simulink model "SOF18d66"  (R2021a)
settings: Solver=VariableStepAuto  StartTime=0.0  StopTime=I_FF.time(end)  RelTol=1e-3
values from neighbouring files (symbols this model uses):
  betapol0 = 0.529567526316    [SOF18d66_setup.mat]
  equilInputs = [0 0 0 0 0 0 0 0 0 0 -1.36186383311e-26 -1.80160126662e-26 ... (15 elements, 1x15)]    [SOF18d66_setup.mat]
  equilOutputs = [-1399.7 -12059 -11927 -3903.5 -12061 -10328 8339.7 10474 2451.8 -17448 -1.80040840482e-24 -2.38174917622e-24 ... (1006 elements, 1x1006)]    [SOF18d66_setup.mat]
  equilVloop = 0.208271873891    [SOF18d66_setup.mat]
  EV_PS =     [SOF18d66_setup.mat]
  Input_struct =     [SOF18d66_setup.mat]
  IV_PS =     [SOF18d66_setup.mat]
  IVC_sat = 1000    [SOF18d66_setup.mat]
  li0 = 0.849401217093    [SOF18d66_setup.mat]
  nCirc = 10    [SOF18d66_setup.mat]
  nGaps = 31    [SOF18d66_setup.mat]
  nInVessel = 2    [SOF18d66_setup.mat]
  nMag = 957    [SOF18d66_setup.mat]
  PFC_sat = [1000 1300 1300 1000 1000 970 970 970 970 1000]    [SOF18d66_setup.mat]
undefined symbols (not defined in the file or in its folder): r_grid, R_grid, VS_contr, z_grid, Z_grid
libraries: cstblocks x6, JT60SA_Magnetic_Control x1
settings Model: Creator=adria  LastModifiedBy=adria

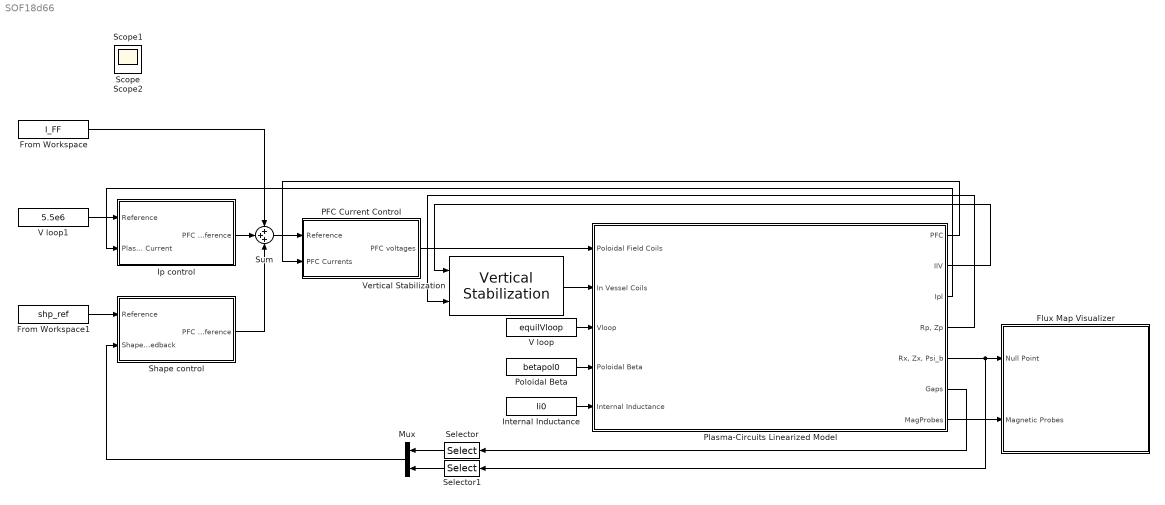
== system SOF18d66 ==
  Flux Map Visualizer : Subsystem  AncestorBlock=JT60SA_Magnetic_Control/Flux Map Visualizer  InitFcn=|  StartFcn=% fig_grid= figure()
      | addpath ./flux_grid_functions
      | [r_grid, z_grid, R_grid, Z_grid, F0, idxGrid] = initFluxGrid(Input_struct,y_np,y_type, mag, 0);
      mask Display:
      | image(['.' filesep 'images' filesep 'Grid.jpg'])
      | port_label('input',1,'Null Point');
      | port_label('input',2, 'Mag Probes');
  From Workspace : FromWorkspace  VariableName=I_FF
  From Workspace1 : FromWorkspace  VariableName=shp_ref
  Internal Inductance : Constant  Value=li0
  Ip control : Subsystem
  Mux : Mux  Inputs=2
  PFC Current Control : Subsystem  AncestorBlock=JT60SA_Magnetic_Control/PFC Current Control
      mask help: PF Coils Current Controller
      mask init:
      | Kpcurr = [5.7832   1.2410        0        0         0       0  0.8592        0        0         0
      |           1.2410   5.7862   1.2432        0         0       0       0        0        0         0
      |                0   1.2432   5.7865   1.2414         0       0       0        0        0         0
      |                0        0   1.2414   5.7845         0       0       0        0        0         0
      |                0        0        0        0   10.9807  2.7576       0        0   0.8679    2.0055
      |                0        0        0        0    2.7576  9.5196  1.2014        0        0         0
      |           0.8592        0        0        0         0  1.2014  6.6407        0        0         0
      |                0        0        0   1.1486         0       0       0  12.5627   2.1557    1.7044
      |                0        0        0        0         0       0       0   2.1557   7.4827    3.7590
      |                0        0        0        0    2.0055       0       0   1.7044   3.7590   14.2743];
  Plasma-Circuits Linearized Model : Subsystem
      mask help: This is an automatically generated block containing a CREATE linearized plasma model. See help for more detailed info on Inputs and Outputs.
      mask Help: The inputs are the voltages on the Poloidal Field Coils, on the In Vessel Coils and on the plasma ring (Vloop), plus the values of poloidal beta and internal inductance The default value of the Vloop is 0. An additional voltage can be inserted, i.e. to simulate the effect of a current drive. The default values of poloidal beta and internal inductance are the equilibrium values; different values can be used to simulate modifications in the plasma profile, and are treated as disturbances by the control systems in the associated library. The available outputs are the currents on the PFC, the IVC, the plasma current,the position of the centroid, the position of the null point and the boundary flux, the fluxes at the magnetic probes and the gaps. The position of the probes and the definition of the gaps can be found in the Input_struct variable, contained in each equilibrium.
      mask Display: image(['.' filesep 'images' filesep 'JT60SA.jpg']);port_label('input', 1, 'PFC Voltages');port_label('input', 2, 'IVC Voltages');port_label('input', 3, 'V_loop');port_label('input', 4, 'Poloidal Beta');port_label('input', 5, 'Internal Inductance');port_label('output', 1, 'PFC Currents');port_label('output', 2, 'IVC Currents');port_label('output', 3, 'Plasma Current');port_label('output', 4, 'Centroid');port_label('output', 5, 'Null Point');port_label('output', 6, 'Gaps');port_label('output', 7, 'Mag Probes');
  Poloidal Beta : Constant  Value=betapol0
  Selector : Selector  InputPortWidth=nGaps  IndexOptions=Index vector (dialog)  Indices=iGap  OutputSizes=1
  Selector1 : Selector  InputPortWidth=3  IndexOptions=Index vector (dialog)  Indices=[1 2]  OutputSizes=1
  Shape control : Subsystem
  Sum : Sum  Inputs=+++
  V loop : Constant  Value=equilVloop
  V loop1 : Constant  Value=5.5e6
  Vertical Stabilization : JT60SA_Magnetic_Control/Vertical Stabilization  Zdot_Gain=VS_contr.d(2)/5.5e6  IVC_Gain=VS_contr.d(1)  VS_Gain=-1
      settings: SourceProductName=JT-60SA Magnetic Control
  Scope : Scope
  Scope1 : Scope
  Scope2 : Scope
  wires:
  V loop/1 -> Plasma-Circuits Linearized Model/3(Vloop)
  Poloidal Beta/1 -> Plasma-Circuits Linearized Model/4(Poloidal Beta)
  Internal Inductance/1 -> Plasma-Circuits Linearized Model/5(Internal Inductance)
  Plasma-Circuits Linearized Model/6(Gaps) -> Selector/1
  Vertical Stabilization/1 -> Plasma-Circuits Linearized Model/2(In Vessel Coils)
  Plasma-Circuits Linearized Model/2(IIV) -> Vertical Stabilization/1
  Plasma-Circuits Linearized Model/4("Rp, Zp") -> Vertical Stabilization/2
  PFC Current Control/1(PFC voltages) -> Plasma-Circuits Linearized Model/1(Poloidal Field Coils)
  Plasma-Circuits Linearized Model/1(PFC) -> PFC Current Control/2(PFC Currents)
  Sum/1 -> PFC Current Control/1(Reference)
  From Workspace/1 -> Sum/1
  Plasma-Circuits Linearized Model/3(Ipl) -> Ip control/2(Plasma Current)
  V loop1/1 -> Ip control/1(Reference)
  Plasma-Circuits Linearized Model/5("Rx, Zx, Psi_b") -> Selector1/1, Flux Map Visualizer/1(Null Point)
  Plasma-Circuits Linearized Model/7(MagProbes) -> Flux Map Visualizer/2(Magnetic Probes)
  From Workspace1/1 -> Shape control/1(Reference)
  Selector/1 -> Mux/1
  Mux/1 -> Shape control/2(Shape feedback)
  Selector1/1 -> Mux/2
  Shape control/1(PFC Currents Reference) -> Sum/3
  Ip control/1(PFC Currents Reference) -> Sum/2

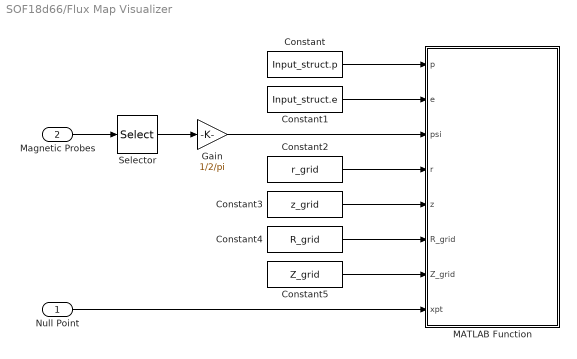
== system SOF18d66/Flux Map Visualizer ==
  Null Point : Inport
  Magnetic Probes : Inport  Port=2
  Constant : Constant  Value=Input_struct.p
  Constant1 : Constant  Value=Input_struct.e
  Constant2 : Constant  Value=r_grid
  Constant3 : Constant  Value=z_grid
  Constant4 : Constant  Value=R_grid
  Constant5 : Constant  Value=Z_grid
  Gain : Gain  Gain=1/2/pi
  MATLAB Function : MATLAB Function  TreatAsAtomicUnit=on  SystemSampleTime=5e-2
  Selector : Selector  InputPortWidth=nMag  IndexOptions=Index vector (dialog)  Indices=idxGrid  OutputSizes=1
  wires:
  Gain/1 -> MATLAB Function/3(psi)
  Null Point/1 -> MATLAB Function/8(xpt)
  Constant5/1 -> MATLAB Function/7(Z_grid)
  Constant4/1 -> MATLAB Function/6(R_grid)
  Constant3/1 -> MATLAB Function/5(z)
  Constant2/1 -> MATLAB Function/4(r)
  Constant1/1 -> MATLAB Function/2(e)
  Constant/1 -> MATLAB Function/1(p)
  Selector/1 -> Gain/1
  Magnetic Probes/1 -> Selector/1

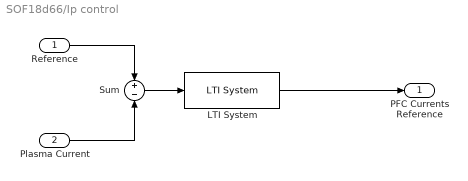
== system SOF18d66/Ip control ==
  Reference : Inport
  Plasma Current : Inport  Port=2
  LTI System : cstblocks/LTI System  sys=Ip_contr  IC=[]
  Sum : Sum  Inputs=+-
  PFC Currents Reference : Outport  VectorParamsAs1DForOutWhenUnconnected=off
  wires:
  Plasma Current/1 -> Sum/2
  Reference/1 -> Sum/1
  LTI System/1 -> PFC Currents Reference/1
  Sum/1 -> LTI System/1

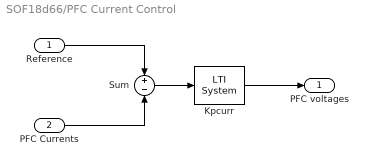
== system SOF18d66/PFC Current Control ==
  Reference : Inport
  PFC Currents : Inport  Port=2
  Kpcurr : cstblocks/LTI System  sys=PF_contr.d  IC=[]
  Sum : Sum  Inputs=+-
  PFC voltages : Outport  VectorParamsAs1DForOutWhenUnconnected=off
  wires:
  Kpcurr/1 -> PFC voltages/1
  Reference/1 -> Sum/1
  PFC Currents/1 -> Sum/2
  Sum/1 -> Kpcurr/1

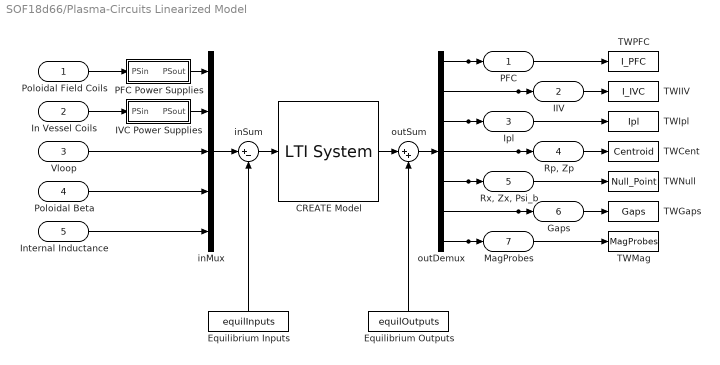
== system SOF18d66/Plasma-Circuits Linearized Model ==
  Poloidal Field Coils : Inport
  In Vessel Coils : Inport  Port=2
  Vloop : Inport  Port=3
  Poloidal Beta : Inport  Port=4
  Internal Inductance : Inport  Port=5
  CREATE Model : cstblocks/LTI System  sys=plasmaStateSpace  IC=[]
  Equilibrium Inputs : Constant  Value=equilInputs
  Equilibrium Outputs : Constant  Value=equilOutputs
  IVC Power Supplies : Subsystem
  PFC Power Supplies : Subsystem
  TWCent : ToWorkspace  VariableName=Centroid  SaveFormat=Structure With Time  SampleTime=-1
  TWGaps : ToWorkspace  VariableName=Gaps  SaveFormat=Structure With Time  SampleTime=-1
  TWIIV : ToWorkspace  VariableName=I_IVC  SaveFormat=Structure With Time  SampleTime=-1
  TWIpl : ToWorkspace  VariableName=Ipl  SaveFormat=Structure With Time  SampleTime=-1
  TWMag : ToWorkspace  VariableName=MagProbes  SaveFormat=Structure With Time  SampleTime=-1
  TWNull : ToWorkspace  VariableName=Null_Point  SaveFormat=Structure With Time  SampleTime=-1
  TWPFC : ToWorkspace  VariableName=I_PFC  SaveFormat=Structure With Time  SampleTime=-1
  inMux : Mux  Inputs=5
  inSum : Sum  Inputs=|+-
  outDemux : Demux  Outputs=[nCirc, nInVessel, 1, 2, 3, nGaps, nMag]
  outSum : Sum  Inputs=|++
  PFC : Outport
  IIV : Outport  Port=2
  Ipl : Outport  Port=3
  "Rp, Zp" : Outport  Port=4
  "Rx, Zx, Psi_b" : Outport  Port=5
  Gaps : Outport  Port=6
  MagProbes : Outport  Port=7
  wires:
  Poloidal Field Coils/1 -> PFC Power Supplies/1(PSin)
  PFC Power Supplies/1(PSout) -> inMux/1
  In Vessel Coils/1 -> IVC Power Supplies/1(PSin)
  IVC Power Supplies/1(PSout) -> inMux/2
  Vloop/1 -> inMux/3
  Poloidal Beta/1 -> inMux/4
  Internal Inductance/1 -> inMux/5
  inMux/1 -> inSum/1
  inSum/1 -> CREATE Model/1
  CREATE Model/1 -> outSum/1
  outSum/1 -> outDemux/1
  outDemux/1 -> PFC/1, TWPFC/1
  outDemux/2 -> IIV/1, TWIIV/1
  outDemux/3 -> Ipl/1, TWIpl/1
  outDemux/4 -> "Rp, Zp"/1, TWCent/1
  outDemux/5 -> "Rx, Zx, Psi_b"/1, TWNull/1
  outDemux/6 -> Gaps/1, TWGaps/1
  outDemux/7 -> MagProbes/1, TWMag/1
  Equilibrium Inputs/1 -> inSum/2
  Equilibrium Outputs/1 -> outSum/2

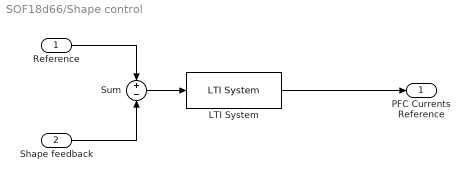
== system SOF18d66/Shape control ==
  Reference : Inport
  Shape feedback : Inport  Port=2
  LTI System : cstblocks/LTI System  sys=SHP_contr  IC=[]
  Sum : Sum  Inputs=+-
  PFC Currents Reference : Outport  VectorParamsAs1DForOutWhenUnconnected=off
  wires:
  Shape feedback/1 -> Sum/2
  Reference/1 -> Sum/1
  LTI System/1 -> PFC Currents Reference/1
  Sum/1 -> LTI System/1

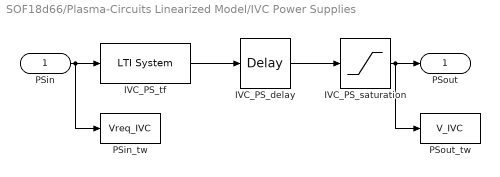
== system SOF18d66/Plasma-Circuits Linearized Model/IVC Power Supplies ==
  PSin : Inport
  IVC_PS_delay : TransportDelay  DelayTime=IV_PS.delay
  IVC_PS_saturation : Saturate  UpperLimit=IVC_sat  LowerLimit=-IVC_sat
  IVC_PS_tf : cstblocks/LTI System  sys=IVC_powerSupply  IC=[]
  PSin_tw : ToWorkspace  VariableName=Vreq_IVC  SaveFormat=Structure With Time
  PSout_tw : ToWorkspace  VariableName=V_IVC  SaveFormat=Structure With Time
  PSout : Outport
  wires:
  PSin/1 -> IVC_PS_tf/1, PSin_tw/1
  IVC_PS_tf/1 -> IVC_PS_delay/1
  IVC_PS_delay/1 -> IVC_PS_saturation/1
  IVC_PS_saturation/1 -> PSout/1, PSout_tw/1

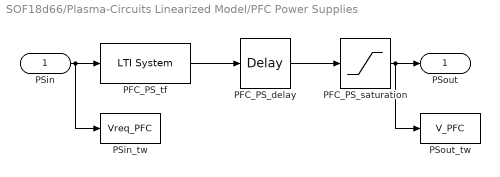
== system SOF18d66/Plasma-Circuits Linearized Model/PFC Power Supplies ==
  PSin : Inport
  PFC_PS_delay : TransportDelay  DelayTime=EV_PS.delay
  PFC_PS_saturation : Saturate  UpperLimit=PFC_sat  LowerLimit=-PFC_sat
  PFC_PS_tf : cstblocks/LTI System  sys=PFC_powerSupply  IC=[]
  PSin_tw : ToWorkspace  VariableName=Vreq_PFC  SaveFormat=Structure With Time
  PSout_tw : ToWorkspace  VariableName=V_PFC  SaveFormat=Structure With Time
  PSout : Outport
  wires:
  PSin/1 -> PFC_PS_tf/1, PSin_tw/1
  PFC_PS_tf/1 -> PFC_PS_delay/1
  PFC_PS_delay/1 -> PFC_PS_saturation/1
  PFC_PS_saturation/1 -> PSout/1, PSout_tw/1

== matlab function SOF18d66/Flux Map Visualizer/MATLAB Function ==
  data: p input; e input; psi input; r input; z input; R_grid input; Z_grid input; xpt input
function plotFluxMap(p,e,psi,r,z,R_grid,Z_grid,xpt)
%#codegen
coder.extrinsic('pdemesh');
coder.extrinsic('fit');
coder.extrinsic('feval');
coder.extrinsic('contour');

psib = xpt(3);

gcf
hold off
h = pdemesh(p,e,[]);
set(h,'Color','black');
axis([0, 6, -4.5, 4.5]), axis equal, hold on

sf = fit([r, z],psi,'linearinterp');      
FF = feval(sf,R_grid,Z_grid);
contour(R_grid,Z_grid,FF, 10);

[~,h] = contour(R_grid,Z_grid,FF, psib*[1 1]);
set(h, 'Color', 'k', 'LineWidth',1.2);

plot(xpt(1), xpt(2), 'ok');
